simulink model "Md61Md62CalibSet"  (R2018b)
settings: Solver=FixedStepDiscrete  StartTime=0.0  StopTime=10.0  FixedStep=0.01  RelTol=1e-3
undefined symbols (not defined in the file or in its folder): KeSMSuFirstRwStBackPosDelta_Val, KeSMSuFirstRwStCushFoldPosDelta_Val, KeSMSuFirstRwStFwdBkwdPosDelta_Val, KeSMSuThrdRwCushFoldPosDelta_Val, KeSMSwAcsMd30PassStBkReclnUpwdDnwdPos1_Val, KeSMSwAcsMd30PassStBkReclnUpwdDnwdPos1Max_Val, KeSMSwAcsMd30PassStBkReclnUpwdDnwdPos1Min_Val, KeSMSwAcsMd30PassStFldUpwdDnwdPos1_Val, KeSMSwAcsMd30PassStFrwdBkwdPos1_Val, KeSMSwAcsMd30PassStFrwdBkwdPos1Max_Val, KeSMSwAcsMd30PassStFrwdBkwdPos1Min_Val, KeSMSwSeatBkLimitPos_Val, KeSMSwSeatBkLimitPosDelt_Val
libraries: StIsPosChkLib x2
(part 5 of 5)

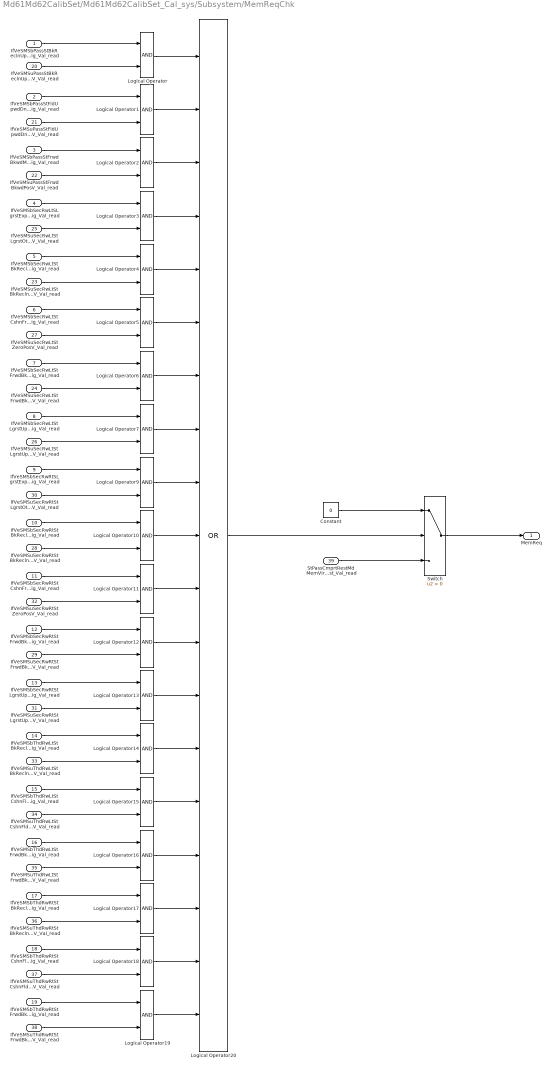
== system Md61Md62CalibSet/Md61Md62CalibSet_Cal_sys/Subsystem/MemReqChk ==
  IfVeSMSbPassStBkReclnUpwdDnwdMovConfig_Val_read : Inport
  IfVeSMSbPassStFldUpwdDnwdMovConfig_Val_read : Inport  Port=2
  IfVeSMSbPassStFrwdBkwdMovConfig_Val_read : Inport  Port=3
  IfVeSMSbSecRwLtSLgrstExpdMovConfig_Val_read : Inport  Port=4
  IfVeSMSbSecRwLtStBkReclnUpwdDnwdMovConfig_Val_read : Inport  Port=5
  IfVeSMSbSecRwLtStCshnFrntUpwdDnwdMovConfig_Val_read : Inport  Port=6
  IfVeSMSbSecRwLtStFrwdBkwdMovConfig_Val_read : Inport  Port=7
  IfVeSMSbSecRwLtStLgrstUpwdMovConfig_Val_read : Inport  Port=8
  IfVeSMSbSecRwRtSLgrstExpdMovConfig_Val_read : Inport  Port=9
  IfVeSMSbSecRwRtStBkReclnUpwdDnwdMovConfig_Val_read : Inport  Port=10
  IfVeSMSbSecRwRtStCshnFrntUpwdDnwdMovConfig_Val_read : Inport  Port=11
  IfVeSMSbSecRwRtStFrwdBkwdMovConfig_Val_read : Inport  Port=12
  IfVeSMSbSecRwRtStLgrstUpwdMovConfig_Val_read : Inport  Port=13
  IfVeSMSbThdRwLtStBkReclnUpwdDnwdMovConfig_Val_read : Inport  Port=14
  IfVeSMSbThdRwLtStCshnFldUpwdDnwdMovConfig_Val_read : Inport  Port=15
  IfVeSMSbThdRwLtStFrwdBkwdMovConfig_Val_read : Inport  Port=16
  IfVeSMSbThdRwRtStBkReclnUpwdDnwdMovConfig_Val_read : Inport  Port=17
  IfVeSMSbThdRwRtStCshnFldUpwdDnwdMovConfig_Val_read : Inport  Port=18
  IfVeSMSbThdRwRtStFrwdBkwdMovConfig_Val_read : Inport  Port=19
  IfVeSMSuPassStBkReclnUpwdDnwdPosV_Val_read : Inport  Port=20
  IfVeSMSuPassStFldUpwdDnwdPosV_Val_read : Inport  Port=21
  IfVeSMSuPassStFrwdBkwdPosV_Val_read : Inport  Port=22
  IfVeSMSuSecRwLtStBkReclnUpwdDnwdPosV_Val_read : Inport  Port=23
  IfVeSMSuSecRwLtStFrwdBkwdPosV_Val_read : Inport  Port=24
  IfVeSMSuSecRwLtStLgrstOtwdInwdPosV_Val_read : Inport  Port=25
  IfVeSMSuSecRwLtStLgrstUpwdDnwdPosV_Val_read : Inport  Port=26
  IfVeSMSuSecRwLtStZeroPosV_Val_read : Inport  Port=27
  IfVeSMSuSecRwRtStBkReclnUpwdDnwdPosV_Val_read : Inport  Port=28
  IfVeSMSuSecRwRtStFrwdBkwdPosV_Val_read : Inport  Port=29
  IfVeSMSuSecRwRtStLgrstOtwdInwdPosV_Val_read : Inport  Port=30
  IfVeSMSuSecRwRtStLgrstUpwdDnwdPosV_Val_read : Inport  Port=31
  IfVeSMSuSecRwRtStZeroPosV_Val_read : Inport  Port=32
  IfVeSMSuThdRwLtStBkReclnUpwdDnwdPosV_Val_read : Inport  Port=33
  IfVeSMSuThdRwLtStCshnFldUpwdDnwdPosV_Val_read : Inport  Port=34
  IfVeSMSuThdRwLtStFrwdBkwdPosV_Val_read : Inport  Port=35
  IfVeSMSuThdRwRtStBkReclnUpwdDnwdPosV_Val_read : Inport  Port=36
  IfVeSMSuThdRwRtStCshnFldUpwdDnwdPosV_Val_read : Inport  Port=37
  IfVeSMSuThdRwRtStFrwdBkwdPosV_Val_read : Inport  Port=38
  StPassCmprtRestMdMemVirtCtrlReqMdadjust_Val_read : Inport  Port=39
  Constant : Constant  Value=0  OutDataTypeStr=uint8
  Logical Operator{,1..7,9..19} (19 alike) : Logic  AllPortsSameDT=off  OutDataTypeStr=boolean
  Logical Operator20 : Logic  Operator=OR  Inputs=19  AllPortsSameDT=off  OutDataTypeStr=boolean
  Switch : Switch  Criteria=u2 > Threshold
  MemReq : Outport
  wires:
  IfVeSMSbPassStBkReclnUpwdDnwdMovConfig_Val_read/1 -> Logical Operator/1
  IfVeSMSbPassStFldUpwdDnwdMovConfig_Val_read/1 -> Logical Operator1/1
  IfVeSMSbPassStFrwdBkwdMovConfig_Val_read/1 -> Logical Operator2/1
  IfVeSMSbSecRwLtSLgrstExpdMovConfig_Val_read/1 -> Logical Operator3/1
  IfVeSMSbSecRwLtStBkReclnUpwdDnwdMovConfig_Val_read/1 -> Logical Operator4/1
  IfVeSMSbSecRwLtStCshnFrntUpwdDnwdMovConfig_Val_read/1 -> Logical Operator5/1
  IfVeSMSbSecRwLtStFrwdBkwdMovConfig_Val_read/1 -> Logical Operator6/1
  IfVeSMSbSecRwLtStLgrstUpwdMovConfig_Val_read/1 -> Logical Operator7/1
  IfVeSMSuPassStBkReclnUpwdDnwdPosV_Val_read/1 -> Logical Operator/2
  IfVeSMSuPassStFldUpwdDnwdPosV_Val_read/1 -> Logical Operator1/2
  IfVeSMSuPassStFrwdBkwdPosV_Val_read/1 -> Logical Operator2/2
  IfVeSMSuSecRwLtStBkReclnUpwdDnwdPosV_Val_read/1 -> Logical Operator4/2
  IfVeSMSuSecRwLtStFrwdBkwdPosV_Val_read/1 -> Logical Operator6/2
  IfVeSMSuSecRwLtStLgrstOtwdInwdPosV_Val_read/1 -> Logical Operator3/2
  IfVeSMSuSecRwLtStLgrstUpwdDnwdPosV_Val_read/1 -> Logical Operator7/2
  IfVeSMSuSecRwLtStZeroPosV_Val_read/1 -> Logical Operator5/2
  IfVeSMSbSecRwRtStBkReclnUpwdDnwdMovConfig_Val_read/1 -> Logical Operator10/1
  IfVeSMSbSecRwRtSLgrstExpdMovConfig_Val_read/1 -> Logical Operator9/1
  IfVeSMSbSecRwRtStCshnFrntUpwdDnwdMovConfig_Val_read/1 -> Logical Operator11/1
  IfVeSMSbSecRwRtStFrwdBkwdMovConfig_Val_read/1 -> Logical Operator12/1
  IfVeSMSbSecRwRtStLgrstUpwdMovConfig_Val_read/1 -> Logical Operator13/1
  IfVeSMSbThdRwLtStBkReclnUpwdDnwdMovConfig_Val_read/1 -> Logical Operator14/1
  IfVeSMSbThdRwRtStFrwdBkwdMovConfig_Val_read/1 -> Logical Operator19/1
  IfVeSMSbThdRwRtStCshnFldUpwdDnwdMovConfig_Val_read/1 -> Logical Operator18/1
  IfVeSMSbThdRwRtStBkReclnUpwdDnwdMovConfig_Val_read/1 -> Logical Operator17/1
  IfVeSMSbThdRwLtStFrwdBkwdMovConfig_Val_read/1 -> Logical Operator16/1
  IfVeSMSbThdRwLtStCshnFldUpwdDnwdMovConfig_Val_read/1 -> Logical Operator15/1
  IfVeSMSuSecRwRtStBkReclnUpwdDnwdPosV_Val_read/1 -> Logical Operator10/2
  IfVeSMSuSecRwRtStFrwdBkwdPosV_Val_read/1 -> Logical Operator12/2
  IfVeSMSuSecRwRtStLgrstOtwdInwdPosV_Val_read/1 -> Logical Operator9/2
  IfVeSMSuSecRwRtStLgrstUpwdDnwdPosV_Val_read/1 -> Logical Operator13/2
  IfVeSMSuSecRwRtStZeroPosV_Val_read/1 -> Logical Operator11/2
  IfVeSMSuThdRwLtStBkReclnUpwdDnwdPosV_Val_read/1 -> Logical Operator14/2
  IfVeSMSuThdRwLtStCshnFldUpwdDnwdPosV_Val_read/1 -> Logical Operator15/2
  IfVeSMSuThdRwLtStFrwdBkwdPosV_Val_read/1 -> Logical Operator16/2
  IfVeSMSuThdRwRtStBkReclnUpwdDnwdPosV_Val_read/1 -> Logical Operator17/2
  IfVeSMSuThdRwRtStCshnFldUpwdDnwdPosV_Val_read/1 -> Logical Operator18/2
  IfVeSMSuThdRwRtStFrwdBkwdPosV_Val_read/1 -> Logical Operator19/2
  Constant/1 -> Switch/1
  StPassCmprtRestMdMemVirtCtrlReqMdadjust_Val_read/1 -> Switch/3
  Logical Operator2/1 -> Logical Operator20/3
  Logical Operator1/1 -> Logical Operator20/2
  Logical Operator/1 -> Logical Operator20/1
  Logical Operator3/1 -> Logical Operator20/4
  Logical Operator4/1 -> Logical Operator20/5
  Logical Operator5/1 -> Logical Operator20/6
  Logical Operator6/1 -> Logical Operator20/7
  Logical Operator7/1 -> Logical Operator20/8
  Logical Operator9/1 -> Logical Operator20/9
  Logical Operator10/1 -> Logical Operator20/10
  Logical Operator11/1 -> Logical Operator20/11
  Logical Operator12/1 -> Logical Operator20/12
  Logical Operator19/1 -> Logical Operator20/19
  Logical Operator18/1 -> Logical Operator20/18
  Logical Operator17/1 -> Logical Operator20/17
  Logical Operator16/1 -> Logical Operator20/16
  Logical Operator15/1 -> Logical Operator20/15
  Logical Operator14/1 -> Logical Operator20/14
  Logical Operator13/1 -> Logical Operator20/13
  Logical Operator20/1 -> Switch/2
  Switch/1 -> MemReq/1
